simulink model "carFollowingSim"  (R2025b)
settings: Solver=VariableStepAuto  StartTime=0.0  StopTime=1000.0  RelTol=1e-3
settings Model: Creator=sprinkle  LastModifiedBy=sprinkle

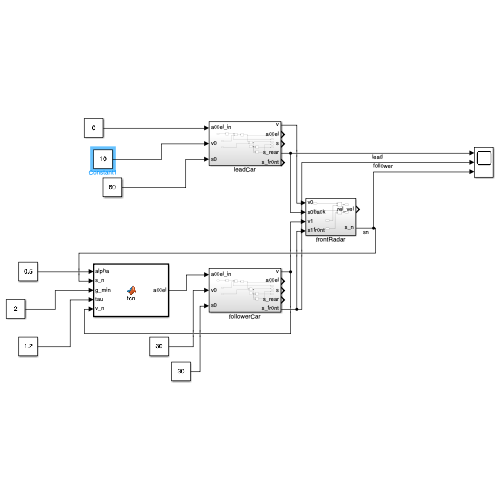
[thumbnail: Simulink's stored preview of the top-level diagram]
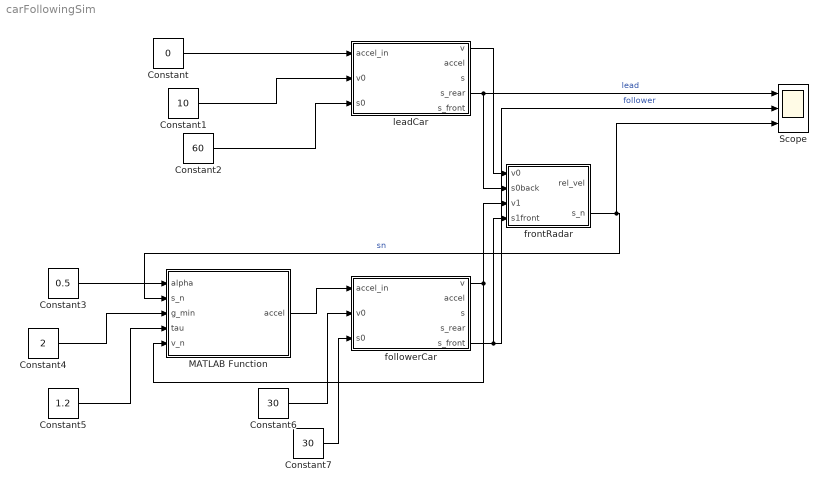
== system carFollowingSim ==
  Constant : Constant  Value=0
  Constant1 : Constant  Value=10
  Constant2 : Constant  Value=60
  Constant3 : Constant  Value=0.5
  Constant4 : Constant  Value=2
  Constant5 : Constant  Value=1.2
  Constant6 : Constant  Value=30
  Constant7 : Constant  Value=30
  MATLAB Function : MATLAB Function  TreatAsAtomicUnit=on
  Scope : Scope  NumInputPorts=3
      settings: ActiveDisplayYMinimum=-38.530882558993781  ActiveDisplayYMaximum=76.005810271346533
  followerCar : Subsystem
  frontRadar : Subsystem
  leadCar : Subsystem
  wires:
  leadCar/1(v) -> frontRadar/1(v0)
  leadCar/4(s_rear) -> Scope/1, frontRadar/2(s0back)  "lead"
  followerCar/1(v) -> frontRadar/3(v1), MATLAB Function/5(v_n)
  followerCar/5(s_front) -> Scope/2, frontRadar/4(s1front)  "follower"
  MATLAB Function/1(accel) -> followerCar/1(accel_in)
  frontRadar/2(s_n) -> Scope/3, MATLAB Function/2(s_n)  "sn"
  Constant1/1 -> leadCar/2(v0)
  Constant2/1 -> leadCar/3(s0)
  Constant/1 -> leadCar/1(accel_in)
  Constant3/1 -> MATLAB Function/1(alpha)
  Constant4/1 -> MATLAB Function/3(g_min)
  Constant5/1 -> MATLAB Function/4(tau)
  Constant7/1 -> followerCar/3(s0)
  Constant6/1 -> followerCar/2(v0)

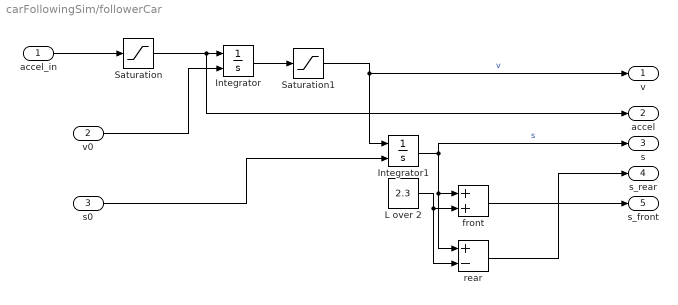
== system carFollowingSim/followerCar ==
  accel_in : Inport
  v0 : Inport  Port=2
  s0 : Inport  Port=3
  Integrator : Integrator  InitialConditionSource=external
  Integrator1 : Integrator  InitialConditionSource=external
  L over 2 : Constant  Value=2.3
  Saturation : Saturate  UpperLimit=1.5  LowerLimit=-3.5
  Saturation1 : Saturate  UpperLimit=30  LowerLimit=0
  front : Sum
  rear : Sum  Inputs=+-
  v : Outport
  accel : Outport  Port=2
  s : Outport  Port=3
  s_rear : Outport  Port=4
  s_front : Outport  Port=5
  wires:
  front/1 -> s_front/1
  s0/1 -> Integrator1/2
  Saturation/1 -> accel/1, Integrator/1
  v0/1 -> Integrator/2
  L over 2/1 -> rear/2, front/2
  Saturation1/1 -> Integrator1/1, v/1  "v"
  rear/1 -> s_rear/1
  accel_in/1 -> Saturation/1
  Integrator/1 -> Saturation1/1
  Integrator1/1 -> s/1, rear/1, front/1  "s"

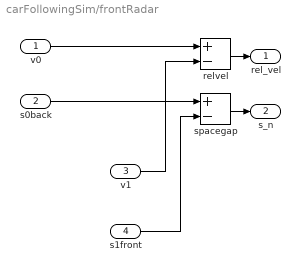
== system carFollowingSim/frontRadar ==
  v0 : Inport
  s0back : Inport  Port=2
  v1 : Inport  Port=3
  s1front : Inport  Port=4
  relvel : Sum  Inputs=+-
  spacegap : Sum  Inputs=+-
  rel_vel : Outport
  s_n : Outport  Port=2
  wires:
  relvel/1 -> rel_vel/1
  s1front/1 -> spacegap/2
  spacegap/1 -> s_n/1
  v0/1 -> relvel/1
  v1/1 -> relvel/2
  s0back/1 -> spacegap/1

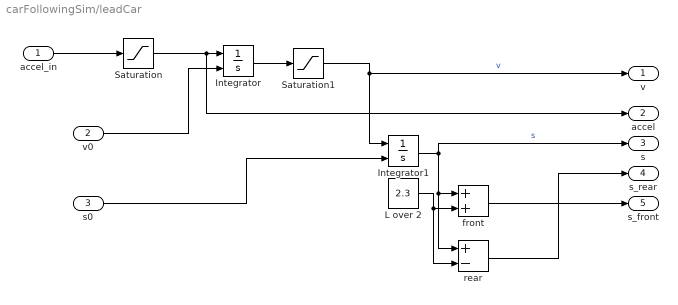
== system carFollowingSim/leadCar ==
  accel_in : Inport
  v0 : Inport  Port=2
  s0 : Inport  Port=3
  Integrator : Integrator  InitialConditionSource=external
  Integrator1 : Integrator  InitialConditionSource=external
  L over 2 : Constant  Value=2.3
  Saturation : Saturate  UpperLimit=1.5  LowerLimit=-3.5
  Saturation1 : Saturate  UpperLimit=30  LowerLimit=0
  front : Sum
  rear : Sum  Inputs=+-
  v : Outport
  accel : Outport  Port=2
  s : Outport  Port=3
  s_rear : Outport  Port=4
  s_front : Outport  Port=5
  wires:
  front/1 -> s_front/1
  s0/1 -> Integrator1/2
  Saturation/1 -> accel/1, Integrator/1
  v0/1 -> Integrator/2
  L over 2/1 -> rear/2, front/2
  Saturation1/1 -> Integrator1/1, v/1  "v"
  rear/1 -> s_rear/1
  accel_in/1 -> Saturation/1
  Integrator/1 -> Saturation1/1
  Integrator1/1 -> s/1, rear/1, front/1  "s"

== matlab function carFollowingSim/MATLAB Function ==
  data: accel output; alpha input; s_n input; g_min input; tau input; v_n input
function accel = fcn(alpha,s_n,g_min,tau,v_n)

accel = alpha*((s_n - g_min) - tau*v_n);
